simulink model "task4"  (R2023a)
settings: Solver=ode23tb  StartTime=0.0  StopTime=25  MaxStep=1e-3  RelTol=1e-3
undefined symbols (not defined in the file): Ion, Lithium
libraries: spsBatteryLib x4, spsIGBTDiodeLib x4, spsSeriesRLCBranchLib x4, spsMosfetLib x2, simulink x1, spsCurrentMeasurementLib x1, spsDCVoltageSourceLib x1, slpidlib x1, spsPWMGeneratorDCDCLib x1, sps_lib x1
settings Model: Creator=gaming3  LastModifiedBy=gaming3

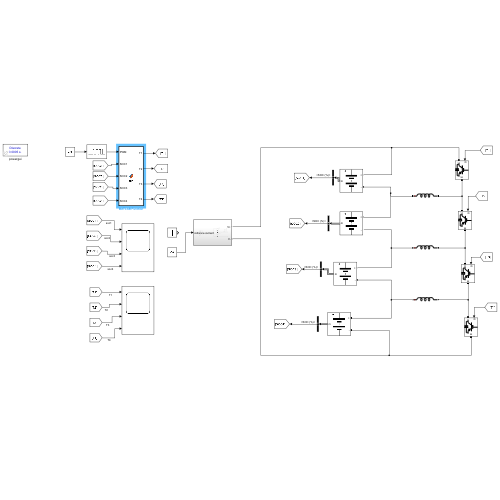
[thumbnail: Simulink's stored preview of the top-level diagram]
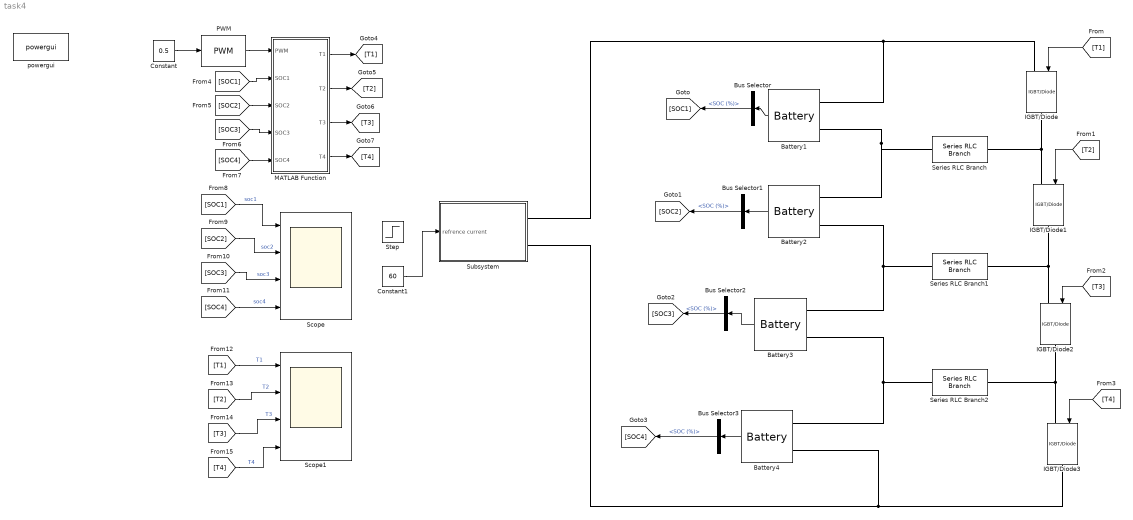
== system task4 ==
  Battery1 : spsBatteryLib/Battery  BatType=Lithium-Ion  ShowTempParam=off  ThermalPreset=no  ShowAgeParam=off  NomV=3.7  NomQ=3.5  SOC=60  Batt_Tr=1  PresetModel=on  MaxQ=3.5  MinV=2.775  FullV=4.3068  Dis_rate=1.5217  R=0.010571  Normal_OP=3.1652  expZone="[3.9974     0.17196]"  current=[6.5 13 32.5]  Units=Time  Tci=20  NomT=20  T2=-30  MaxQ2=4.8  FullV2=7.1  Normal_OP2=5.655  expZone2="[6.58           1]"  Rca=0.6  ti=2000  Dp=0  Neq0=0  Tsim=1e6  Ta1=25  Qeol=5.4*0.9  Reol=0.013333*1.2  Char_age=[2.3478, 3]  Dis_age=[2.3478, 10]  N1=1500  N2=10500  N3=1000  N4=1400  Ta2=45  N5=950
  Battery2 : spsBatteryLib/Battery  BatType=Lithium-Ion  ShowTempParam=off  ThermalPreset=no  ShowAgeParam=off  NomV=3.9  NomQ=4  SOC=40  Batt_Tr=1  PresetModel=on  MaxQ=4  MinV=2.925  FullV=4.5395  Dis_rate=1.7391  R=0.00975  Normal_OP=3.6174  expZone="[4.2135     0.19652]"  current=[6.5 13 32.5]  Units=Time  Tci=20  NomT=20  T2=-30  MaxQ2=4.8  FullV2=7.1  Normal_OP2=5.655  expZone2="[6.58           1]"  Rca=0.6  ti=2000  Dp=0  Neq0=0  Tsim=1e6  Ta1=25  Qeol=5.4*0.9  Reol=0.013333*1.2  Char_age=[2.3478, 3]  Dis_age=[2.3478, 10]  N1=1500  N2=10500  N3=1000  N4=1400  Ta2=45  N5=950
  Battery3 : spsBatteryLib/Battery  BatType=Lithium-Ion  ShowTempParam=off  ThermalPreset=no  ShowAgeParam=off  NomV=3.7  NomQ=3.7  SOC=55  Batt_Tr=1  PresetModel=on  MaxQ=3.7  MinV=2.775  FullV=4.3068  Dis_rate=1.6087  R=0.01  Normal_OP=3.3461  expZone="[3.9974     0.18178]"  current=[6.5 13 32.5]  Units=Time  Tci=20  NomT=20  T2=-30  MaxQ2=4.8  FullV2=7.1  Normal_OP2=5.655  expZone2="[6.58           1]"  Rca=0.6  ti=2000  Dp=0  Neq0=0  Tsim=1e6  Ta1=25  Qeol=5.4*0.9  Reol=0.013333*1.2  Char_age=[2.3478, 3]  Dis_age=[2.3478, 10]  N1=1500  N2=10500  N3=1000  N4=1400  Ta2=45  N5=950
  Battery4 : spsBatteryLib/Battery  BatType=Lithium-Ion  ShowTempParam=off  ThermalPreset=no  ShowAgeParam=off  NomV=4  NomQ=4  SOC=49  Batt_Tr=1  PresetModel=on  MaxQ=4  MinV=3  FullV=4.6559  Dis_rate=1.7391  R=0.01  Normal_OP=3.6174  expZone="[4.3215     0.19652]"  current=[6.5 13 32.5]  Units=Time  Tci=20  NomT=20  T2=-30  MaxQ2=4.8  FullV2=7.1  Normal_OP2=5.655  expZone2="[6.58           1]"  Rca=0.6  ti=2000  Dp=0  Neq0=0  Tsim=1e6  Ta1=25  Qeol=5.4*0.9  Reol=0.013333*1.2  Char_age=[2.3478, 3]  Dis_age=[2.3478, 10]  N1=1500  N2=10500  N3=1000  N4=1400  Ta2=45  N5=950
  Bus Selector{,1..3} (4 alike) : BusSelector  OutputSignals=SOC (%)
  Constant : Constant  Value=0.5
  Constant1 : Constant  Value=60
  IGBT/Diode{,1..3} (4 alike) : spsIGBTDiodeLib/IGBT//Diode  Ron=1e-3  Rs=1e5  Cs=inf  Measurements=off
  MATLAB Function : MATLAB Function  TreatAsAtomicUnit=on
  PWM : simulink/Discontinuities/PWM  DisableCoverage=on  Period=1/10e3  InitialDelay=0  DisallowZeroDutyCycle=off  RunAtFixedTimeIntervals=off  SampleTime=0.1
  Scope : Scope  NumInputPorts=4
  Scope1 : Scope  NumInputPorts=4
  Series RLC Branch : spsSeriesRLCBranchLib/Series RLC Branch  LConnTagsString=__new0  RConnTagsString=__new0  BranchType=L  Resistance=1  Inductance=1e-3  SetiL0=off  InitialCurrent=0  Capacitance=1e-6  Setx0=off  InitialVoltage=0  Measurements=None
  Series RLC Branch1 : spsSeriesRLCBranchLib/Series RLC Branch  LConnTagsString=__new0  RConnTagsString=__new0  BranchType=L  Resistance=1  Inductance=1e-3  SetiL0=off  InitialCurrent=0  Capacitance=1e-6  Setx0=off  InitialVoltage=0  Measurements=None
  Series RLC Branch2 : spsSeriesRLCBranchLib/Series RLC Branch  LConnTagsString=__new0  RConnTagsString=__new0  BranchType=L  Resistance=1  Inductance=1e-3  SetiL0=off  InitialCurrent=0  Capacitance=1e-6  Setx0=off  InitialVoltage=0  Measurements=None
  Step : Step  Time=5  Before=60  After=-60  SampleTime=0
  Subsystem : Subsystem
  powergui : sps_lib/powergui  Priority=1  SimulationMode=Discrete  SampleTime=0.0005  frequency=60  Iterations=50  frequencyindice=0  Pbase=100e6  ErrMax=1e-4  UnitsV=kV  UnitsW=MW  buscounter=0  FunctionMessages=off  echomessages=off  EnableUseOfTLC=off  CurrentSourceSwitches=off  DisableSnubberDevices=off  DisableRonSwitches=off  DisableVfSwitches=off  DisplayEquations=off  AutomaticDiscreteSolvers=off  SolverType=Tustin/Backward Euler (TBE)  Interpol=off  ExternalGateDelay=off  methode=off  Ts=100  x0status=blocks  SPID=on  SwTol=0  HookPort=off  NonlinearTolerance=1e-4  nMaxIteration=100  ContinueOnMaxIteration=off  RestoreLinks=warning  ResistiveCurrentMeasurement=off  Frange=[0:2:500]  Ylog=off  Xlog=on  ShowGrid=off  save=off  variable=ZData  structure=0  ZoomFFT=off  StartTime=0.0  cycles=1  DisplayStyle=1  fundamental=60  FreqAxis=off  MaxFrequency=1000  frequencyindicesteady=1  RmsSteady=1  display=off
  wires:
  [T1] -> IGBT/Diode/1
  [SOC1] -> Scope/1  "soc1"
  Constant/1 -> PWM/1
  [SOC1] -> MATLAB Function/2(SOC1)
  [SOC2] -> MATLAB Function/3(SOC2)
  [SOC3] -> MATLAB Function/4(SOC3)
  [T1] -> Scope1/1  "T1"
  Battery3/1 -> Bus Selector2/1
  Bus Selector3/1 -> [SOC4]  "<SOC (%)>"
  [SOC4] -> MATLAB Function/5(SOC4)
  Bus Selector/1 -> [SOC1]  "<SOC (%)>"
  [T3] -> Scope1/3  "T3"
  MATLAB Function/2(T2) -> [T2]
  Bus Selector2/1 -> [SOC3]  "<SOC (%)>"
  MATLAB Function/1(T1) -> [T1]
  [SOC2] -> Scope/2  "soc2"
  [T4] -> IGBT/Diode3/1
  [SOC4] -> Scope/4  "soc4"
  MATLAB Function/4(T4) -> [T4]
  [T4] -> Scope1/4  "T4"
  Battery1/1 -> Bus Selector/1
  Battery4/1 -> Bus Selector3/1
  PWM/1 -> MATLAB Function/1(PWM)
  [T2] -> Scope1/2  "T2"
  [SOC3] -> Scope/3  "soc3"
  [T2] -> IGBT/Diode1/1
  Bus Selector1/1 -> [SOC2]  "<SOC (%)>"
  MATLAB Function/3(T3) -> [T3]
  Battery2/1 -> Bus Selector1/1
  [T3] -> IGBT/Diode2/1
  Constant1/1 -> Subsystem/1(refrence current)
  connections:
  Series RLC Branch/LConn1 -- Battery1/LConn2 -- Battery2/LConn1
  Series RLC Branch2/RConn1 -- IGBT/Diode3/LConn1 -- IGBT/Diode2/RConn1
  Battery3/LConn2 -- Battery4/LConn1 -- Series RLC Branch2/LConn1
  Series RLC Branch/RConn1 -- IGBT/Diode/RConn1 -- IGBT/Diode1/LConn1
  Subsystem/RConn1 -- IGBT/Diode/LConn1 -- Battery1/LConn1
  Series RLC Branch1/LConn1 -- Battery2/LConn2 -- Battery3/LConn1
  Series RLC Branch1/RConn1 -- IGBT/Diode1/RConn1 -- IGBT/Diode2/LConn1
  Battery4/LConn2 -- IGBT/Diode3/RConn1 -- Subsystem/RConn2

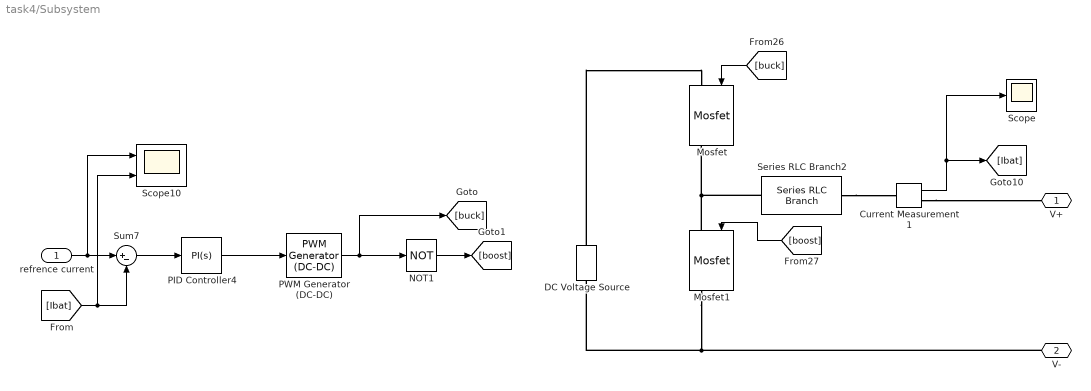
== system task4/Subsystem ==
  refrence current : Inport
  Current Measurement1 : spsCurrentMeasurementLib/Current Measurement  PhasorSimulation=off  OutputType=Complex  PSBequivalent=0
  DC Voltage Source : spsDCVoltageSourceLib/DC Voltage Source  Amplitude=100  Measurements=None
  Mosfet : spsMosfetLib/Mosfet  Ron=0.1  Lon=0  Rd=0.01  Vfd=0  IC=0  Rs=1e5  Cs=inf  Measurements=on
  Mosfet1 : spsMosfetLib/Mosfet  Ron=0.1  Lon=0  Rd=0.01  Vfd=0  IC=0  Rs=1e5  Cs=inf  Measurements=on
  NOT1 : Logic  Operator=NOT  IconShape=distinctive  AllPortsSameDT=off  OutDataTypeStr=boolean
  PID Controller4 : slpidlib/PID Controller  Controller=PI  Form=Parallel  TimeDomain=Continuous-time  UseExternalTs=off  SampleTime=-1  IntegratorMethod=Forward Euler  FilterMethod=Forward Euler  ControllerParametersSource=internal  P=500  I=1000  UseKiTs=off  D=0  N=100  UseFilter=on  TunerSelectOption=Transfer Function Based (PID Tuner App)  InitialConditionSource=internal  InitialConditionForIntegrator=0  InitialConditionForFilter=0  DifferentiatorICPrevScaledInput=0  ExternalReset=none  TrackingMode=off  Kt=1  LimitOutput=on  SatLimitsSource=internal  UpperSaturationLimit=0.95  LowerSaturationLimit=0  LinearizeAsGain=on  AntiWindupMode=clamping  Kb=1  LimitIntegrator=off  UpperIntegratorSaturationLimit=inf  LowerIntegratorSaturationLimit=-inf  POutMin=[]  POutMax=[]  IOutMin=[]  IOutMax=[]  DOutMin=[]  DOutMax=[]  NOutMin=[]  NOutMax=[]  SumOutMin=[]  SumOutMax=[]  SaturationOutMin=[]  SaturationOutMax=[]  PParamMin=[]  PParamMax=[]  IParamMin=[]  IParamMax=[]  DParamMin=[]  DParamMax=[]  NParamMin=[]  NParamMax=[]  KbParamMin=[]  KbParamMax=[]  KtParamMin=[]  KtParamMax=[]  KbOutMin=[]  KbOutMax=[]  KtOutMin=[]  KtOutMax=[]  IntegratorOutMin=[]  IntegratorOutMax=[]  FilterOutMin=[]  FilterOutMax=[]  SumI1OutMin=[]  SumI1OutMax=[]  SumI2OutMin=[]  SumI2OutMax=[]  SumI3OutMin=[]  SumI3OutMax=[]  SumI4OutMin=[]  SumI4OutMax=[]  SumDOutMin=[]  SumDOutMax=[]  DifferentiatorOutMin=[]  DifferentiatorOutMax=[]  FilterDiffOutCoefMin=[]  FilterDiffOutCoefMax=[]  ReciprocalOutMin=[]  ReciprocalOutMax=[]  SumDenOutMin=[]  SumDenOutMax=[]  SumNumOutMin=[]  SumNumOutMax=[]  DivideOutMin=[]  DivideOutMax=[]  UdiffTsProdOutMin=[]  UdiffTsProdOutMax=[]  NTsProdOutMin=[]  NTsProdOutMax=[]  UintegralTsProdOutMin=[]  UintegralTsProdOutMax=[]  UngainTsProdOutMin=[]  UngainTsProdOutMax=[]  ClampingZeroOutDataTypeStr=Inherit: Inherit via back propagation  ClampingZeroOutMin=[]  ClampingZeroOutMax=[]  FilterDenConstantOutDataTypeStr=Inherit: Inherit via back propagation  FilterDenConstantOutMin=[]  FilterDenConstantOutMax=[]  PCopyOutDataTypeStr=Inherit: Inherit via back propagation  PCopyOutMin=[]  PCopyOutMax=[]  NCopyOutDataTypeStr=Inherit: Inherit via back propagation  NCopyOutMin=[]  NCopyOutMax=[]  IntegratorContinuousStateAttributes=''  IntegratorStateMustResolveToSignalObject=off  IntegratorRTWStateStorageClass=Auto  FilterContinuousStateAttributes=''  FilterStateMustResolveToSignalObject=off  FilterRTWStateStorageClass=Auto  ParallelPVariant=InternalParameters  IdealPVariant=Disabled  IVariant=InternalParameters  DVariant=Disabled  IntegratorVariant=Continuous  SatVariant=Enabled  AWVariant=ContClampingParallel  PCopyVariant=Disabled  TRVariant=Disabled  FdbkBlocksVariant=Forward  IdealPFdbkVariant=Disabled  SatFdbkVariant=Disabled  DerivativeFilterVariant=Disabled  NVariant=Disabled  NCopyVariant=Disabled_SignalSpec  FilterICVariant=Disabled  IntegratorICVariant=InternalICs  ExternalResetVariant=Disabled  TRSumVariant=Passthrough  SumFdbkVariant=Disabled  SumVariant=Sum_PI  TsampFilterVariant=InternalTs  TsampNgainVariant=Passthrough  TsampIntegralVariant=Disabled_SignalSpec  ExternalSaturationOutDataTypeStr=Inherit: Same as second input
  PWM Generator (DC-DC) : spsPWMGeneratorDCDCLib/PWM Generator (DC-DC)  Fsw=5000  Ts=0
  Scope : Scope
  Scope10 : Scope  NumInputPorts=2
  Series RLC Branch2 : spsSeriesRLCBranchLib/Series RLC Branch  LConnTagsString=__new0  RConnTagsString=__new0  BranchType=L  Resistance=1  Inductance=0.01536  SetiL0=off  InitialCurrent=0  Capacitance=1e-6  Setx0=off  InitialVoltage=0  Measurements=None
  Sum7 : Sum  Inputs=|+-
  V+ : PMIOPort  Side=Right
  V- : PMIOPort  Port=2  Side=Right
  wires:
  [Ibat] -> Scope10/2, Sum7/2
  refrence current/1 -> Scope10/1, Sum7/1
  PWM Generator (DC-DC)/1 -> [buck], NOT1/1
  [boost] -> Mosfet1/1
  [buck] -> Mosfet/1
  Current Measurement1/1 -> Scope/1, [Ibat]
  NOT1/1 -> [boost]
  Sum7/1 -> PID Controller4/1
  PID Controller4/1 -> PWM Generator (DC-DC)/1
  connections:
  Series RLC Branch2/RConn1 -- Current Measurement1/LConn1
  Series RLC Branch2/LConn1 -- Mosfet/RConn1 -- Mosfet1/LConn1
  DC Voltage Source/RConn1 -- Mosfet/LConn1
  Current Measurement1/RConn1 -- V+/RConn1
  DC Voltage Source/LConn1 -- V-/RConn1 -- Mosfet1/RConn1

== matlab function task4/MATLAB Function ==
  data: PWM input; T1 output; T2 output; T3 output; SOC1 input; SOC2 input; SOC3 input; T4 output; SOC4 input
function [T1,T2,T3,T4] = fcn(PWM, SOC1, SOC2, SOC3, SOC4)

persistent balancing_active

if isempty(balancing_active)
    balancing_active = false;
end

SOC = [SOC1, SOC2, SOC3, SOC4];
SOC_diff = max(SOC) - min(SOC);

% Apply hysteresis logic
if ~balancing_active && SOC_diff > 5
    balancing_active = true;
elseif balancing_active && SOC_diff <= 3
    balancing_active = false;
end

if balancing_active
    T = (SOC > min(SOC)) * PWM;  % Balance: only cells with SOC > min get PWM
else
    T = zeros(1, 4);  % No balancing
end

[T1, T2, T3, T4] = deal(T(1), T(2), T(3), T(4));
end
